simulink model "PubIfDecisionTOS_MDL"  (R2020b)
settings: configuration reference "DspaceConfig" (kept outside this file)
PostLoadFcn:
  | if any(exist('dsrtsu_mdlpostloadfcn', 'file') ~= 0), dsrtsu_mdlpostloadfcn('Execute', bdroot); end
InitFcn:
  | , if any(exist('dsmpb_private', 'file') ~= 0), dsmpb_private('dsmpb_mdlclblib', 'Init', bdroot); end,
undefined symbols (not defined in the file or in its folder): C_TOS_ACCEgoRAxletoFbumplength_m, C_TOS_ACCTargetFront_Flag, C_TOS_AEBJAPedObjDxThre_Val, C_TOS_AEBJAPedObjDyThre_Val, C_TOS_AEBJATargetSize_Val, C_TOS_AEBJAVehObjDxThre_Val, C_TOS_AEBJAVehObjDyThre_Val, C_TOS_AEBJuncPedTargetSize_Val, C_TOS_AEBLatObjDxThre_Val, C_TOS_AEBLatPedDyThre_Val, C_TOS_AEBLatTargetSize_Val, C_TOS_AEBLongTargetInEgoFront_Flag, C_TOS_axAbsGround_Parameter, C_TOS_CameraConfirmedFlag, C_TOS_CNsubjWidth, C_TOS_CurrentLaneCoreMinWidth_Val, C_TOS_CutInProb_Val_Zero, C_TOS_CutOutProb_Val_Zero, C_TOS_D2R_Val, C_TOS_DefaultValueObjectToCenterLine_dy, C_TOS_EgoCarWidth_Val, C_TOS_EgoDxRefPoint_m, C_TOS_EgoRAxletoFbumplength_m, C_TOS_HalfWidthVehicle_Con, C_TOS_HWA_CurrentLaneFlag, C_TOS_HWA_LeftLaneFlag, C_TOS_HWA_MovingDir_Vaild, C_TOS_HWA_MovState_Vaild, C_TOS_HWA_RightLaneFlag, C_TOS_LaneLineCourseErrorFront, C_TOS_LaneLineCourseErrorRear, C_TOS_MotorbikeDefaultWidth_m, C_TOS_NumberOfEffectiveTargets, C_TOS_Obj_Age_Val, C_TOS_Objdx_Constraint_Val, C_TOS_ObjectDefaultWidth_m, C_TOS_ObjInCurrentLane_Val, C_TOS_ObjInCurrentLaneValid, C_TOS_ObjInLeftLaneValid, C_TOS_ObjInRightLaneValid, C_TOS_ObjNotInCurrentLane_Val, C_TOS_ObjNotREElementType, C_TOS_ObjPredictDis_dy_ConstantVal_Zeros, C_TOS_ObjToCenterLine_ConstantVal_Zeros, C_TOS_OFMObjIDInvilad_Val, C_TOS_PIL_LatDisCons_Val_zero, C_TOS_PIL_ObjectCutInFlag_b, C_TOS_PIL_ObjectCutOutFlag_b, C_TOS_PIL_ObjLaneProb_al_Val, C_TOS_PP_ObjFusType_FC_Confirm_b, C_TOS_PP_ObjFusType_FC_FR_Confirm_b, C_TOS_PP_ObjFusType_FR_Confirm_b, C_TOS_RE_80BoolDefault_Val, C_TOS_RE_80Single181Default_Val, C_TOS_RE_80Single255Default_Val, C_TOS_RE_80Uint8Default_Val, C_TOS_RE_D2R, C_TOS_RE_D_180_Val, C_TOS_RE_InvalidObjectID_Val, C_TOS_RE_InvalidTargetChainDir_Val ... (+142)
libraries: simulink x1650, TOS_LIB x361, canfdmsglib x14
(part 30 of 69)

== system PubIfDecisionTOS_MDL/TOS_20201112/TOS_2012080320/TOS/LC_LCKie_ELK/TOS_HWA/CurrentLane/HWA_CurrentLane_Target/HWA_CLF_Target_1 ==
  HWA_CLF_Trg_1_Index : Inport
  Object_ID : Inport  Port=2
  Object_Fus_Type : Inport  Port=3
  object_MovingState : Inport  Port=4
  PP_ObjMovingDirSignalProcessing : Inport  Port=5
  Object_HeadingAngle : Inport  Port=6
  Object_DX : Inport  Port=7
  TOS_TLJ_SameLaneConfirm_Flag : Inport  Port=8
  Object_Type : Inport  Port=9
  Object_ObstacleProb : Inport  Port=10
  Object_DY : Inport  Port=11
  PP_ObjFusType_FC_FR_Confirm : Inport  Port=12
  PP_ObjFusType_FR_Confirm : Inport  Port=13
  PP_ObjFusType_FC_Confirm : Inport  Port=14
  Object_VX : Inport  Port=15
  Object_VY : Inport  Port=16
  VIE_EgoVelocity : Inport  Port=17
  SteerWheelAng : Inport  Port=18
  PIL_OverlapRatio : Inport  Port=19
  HWA_CLF_Target_ID_K1 : Inport  Port=20
  HWA_CLF_Target_ID_K2 : Inport  Port=21
  HWA_CLF_Target_MovState_K1 : Inport  Port=22
  HWA_CLF_Target_MovState_K2 : Inport  Port=23
  LM_LR_Line04_dDisStart : Inport  Port=24
  LM_LR_Line04_dDisEnd : Inport  Port=25
  LM_LR_Line05_dDisStart : Inport  Port=26
  LM_LR_Line05_dDisEnd : Inport  Port=27
  LM_LR_Line06_dDisStart : Inport  Port=28
  LM_LR_Line06_dDisEnd : Inport  Port=29
  LM_LR_Line04_pC2 : Inport  Port=30
  LM_LR_Line05_pC2 : Inport  Port=31
  LM_LR_Line06_pC2 : Inport  Port=32
  LM_LR_Line04_fCamValid : Inport  Port=33
  LM_LR_Line05_fCamValid : Inport  Port=34
  LM_LR_Line06_fCamValid : Inport  Port=35
  LM_LR_Line04_pC0 : Inport  Port=36
  LM_RL_Line04_pC0 : Inport  Port=37
  Compare To Constant : simulink/Logic and Bit Operations/Compare To Constant  relop===  const=C_TOS_OFMObjIDInvilad_Val  OutDataTypeStr=boolean
      settings: AttributesFormatString=C_TOS_OFMObjIDInvilad_Val = 0
  Constant1 : Constant  Value=0  OutDataTypeStr=uint8
  HWA_CLF_Target : Subsystem
  HWA_CLF_TargetDefault : Subsystem  TreatAsAtomicUnit=on
  If : If  IfExpression=u1 ~= 0
  Merge{,1..18} (19 alike) : Merge
  Selector3 : Selector  InputPortWidth=3  IndexOptions=Index vector (dialog)  Indices=1  OutputSizes=1
  Switch1 : Switch  Criteria=u2 ~= 0
  HWA_CLF_Target_1_Index : Outport
  HWA_CLF_Target_FusionType_ObserVale : Outport  Port=2
  HWA_CLF_Target_TrgMovDir_ObserVale : Outport  Port=3
  HWA_CLF_Target_TargetDxConfirm_ObserVale : Outport  Port=4
  HWA_CLF_Target_ObjType_ObserVale : Outport  Port=5
  HWA_CLF_Target_ObstacleProb_ObserVale : Outport  Port=6
  HWA_CLF_Target_DyConfirm_ObserVale : Outport  Port=7
  HWA_CLF_Target_TrgMovDirFlag_1_ObserVale : Outport  Port=8
  HWA_CLF_Target_TrgMovDirFlag_2_ObserVale : Outport  Port=9
  HWA_CLF_Target_TrgMovDirFlag_3_ObserVale : Outport  Port=10
  HWA_CLF_Target_TrgMovDirFlag_4_ObserVale : Outport  Port=11
  HWA_CLF_Target_TrgMovDirFlag_5_ObserVale : Outport  Port=12
  HWA_CLF_Target_TrgMovDirFlag_6_ObserVale : Outport  Port=13
  HWA_CLF_Target_DyConfirm_1_ObserVale : Outport  Port=14
  HWA_CLF_Target_DyConfirm_2_ObserVale : Outport  Port=15
  HWA_CLF_Target_DyConfirm_3_ObserVale : Outport  Port=16
  HWA_CLF_Target_DyConfirm_4_OverlapRatio_ObserVale : Outport  Port=17
  HWA_CLF_Target_DyConfirm_5_OverlapConfirm_ObserVale : Outport  Port=18
  HWA_CLF_Target_DyConfirm_ALL_6_ObserVale : Outport  Port=19
  wires:
  LM_RL_Line04_pC0/1 -> HWA_CLF_Target/37(LM_RL_Line04_pC0)  "LM_RL_Line04_pC0"
  LM_LR_Line04_pC0/1 -> HWA_CLF_Target/36(LM_LR_Line04_pC0)  "LM_LR_Line04_pC0"
  HWA_CLF_TargetDefault/19(HWA_CLF_Target_DyConfirm_ALL_6_ObserVale) -> Merge18/1
  Merge18/1 -> HWA_CLF_Target_DyConfirm_ALL_6_ObserVale/1
  HWA_CLF_Target/19(HWA_CLF_Target_DyConfirm_ALL_6_ObserVale) -> Merge18/2
  HWA_CLF_TargetDefault/18(HWA_CLF_Target_DyConfirm_5_OverlapConfirm_ObserVale) -> Merge17/1
  HWA_CLF_TargetDefault/17(HWA_CLF_Target_DyConfirm_4_OverlapRatio_ObserVale) -> Merge15/1
  HWA_CLF_TargetDefault/16(HWA_CLF_Target_DyConfirm_3_ObserVale) -> Merge14/1
  HWA_CLF_TargetDefault/15(HWA_CLF_Target_DyConfirm_2_ObserVale) -> Merge13/1
  HWA_CLF_TargetDefault/14(HWA_CLF_Target_DyConfirm_1_ObserVale) -> Merge16/1
  HWA_CLF_TargetDefault/13(HWA_CLF_Target_TrgMovDirFlag_6_ObserVale) -> Merge8/1
  HWA_CLF_TargetDefault/12(HWA_CLF_Target_TrgMovDirFlag_5_ObserVale) -> Merge12/1
  HWA_CLF_TargetDefault/11(HWA_CLF_Target_TrgMovDirFlag_4_ObserVale) -> Merge11/1
  HWA_CLF_TargetDefault/10(HWA_CLF_Target_TrgMovDirFlag_3_ObserVale) -> Merge10/1
  HWA_CLF_TargetDefault/9(HWA_CLF_Target_TrgMovDirFlag_2_ObserVale) -> Merge9/1
  HWA_CLF_TargetDefault/8(HWA_CLF_Target_TrgMovDirFlag_1_ObserVale) -> Merge7/1
  HWA_CLF_TargetDefault/7(HWA_CLF_Target_DyConfirm_ObserVale) -> Merge6/1
  HWA_CLF_TargetDefault/6(HWA_CLF_Target_ObstacleProb_ObserVale) -> Merge5/1
  HWA_CLF_TargetDefault/5(HWA_CLF_Target_ObjType_ObserVale) -> Merge4/1
  HWA_CLF_TargetDefault/4(HWA_CLF_Target_TargetDxConfirm_ObserVale) -> Merge3/1
  HWA_CLF_TargetDefault/3(HWA_CLF_Target_TrgMovDir_ObserVale) -> Merge2/1
  HWA_CLF_TargetDefault/2(HWA_CLF_Target_FusionType_ObserVale) -> Merge1/1
  HWA_CLF_TargetDefault/1(HWA_CLF_Target_2_TargeConfirm) -> Merge/1
  HWA_CLF_Target/18(HWA_CLF_Target_DyConfirm_5_OverlapConfirm_ObserVale) -> Merge17/2
  Merge17/1 -> HWA_CLF_Target_DyConfirm_5_OverlapConfirm_ObserVale/1
  LM_LR_Line06_fCamValid/1 -> HWA_CLF_Target/35(LM_LR_Line06_fCamValid)
  LM_LR_Line05_fCamValid/1 -> HWA_CLF_Target/34(LM_LR_Line05_fCamValid)
  LM_LR_Line04_fCamValid/1 -> HWA_CLF_Target/33(LM_LR_Line04_fCamValid)
  LM_LR_Line06_pC2/1 -> HWA_CLF_Target/32(LM_LR_Line06_pC2)
  LM_LR_Line05_pC2/1 -> HWA_CLF_Target/31(LM_LR_Line05_pC2)
  LM_LR_Line04_pC2/1 -> HWA_CLF_Target/30(LM_LR_Line04_pC2)
  LM_LR_Line06_dDisEnd/1 -> HWA_CLF_Target/29(LM_LR_Line06_dDisEnd)
  LM_LR_Line06_dDisStart/1 -> HWA_CLF_Target/28(LM_LR_Line06_dDisStart)
  LM_LR_Line05_dDisEnd/1 -> HWA_CLF_Target/27(LM_LR_Line05_dDisEnd)
  LM_LR_Line05_dDisStart/1 -> HWA_CLF_Target/26(LM_LR_Line05_dDisStart)
  LM_LR_Line04_dDisEnd/1 -> HWA_CLF_Target/25(LM_LR_Line04_dDisEnd)
  LM_LR_Line04_dDisStart/1 -> HWA_CLF_Target/24(LM_LR_Line04_dDisStart)
  HWA_CLF_Target/14(HWA_CLF_Target_DyConfirm_1_ObserVale) -> Merge16/2
  Merge16/1 -> HWA_CLF_Target_DyConfirm_1_ObserVale/1
  Switch1/1 -> HWA_CLF_Target_1_Index/1
  Selector3/1 -> [HWA_CurrentFront_Target_1_Index], Compare To Constant/1
  Merge15/1 -> HWA_CLF_Target_DyConfirm_4_OverlapRatio_ObserVale/1
  Merge14/1 -> HWA_CLF_Target_DyConfirm_3_ObserVale/1
  Merge13/1 -> HWA_CLF_Target_DyConfirm_2_ObserVale/1
  HWA_CLF_Target/17(HWA_CLF_Target_DyConfirm_4_OverlapRatio_ObserVale) -> Merge15/2
  HWA_CLF_Target/16(HWA_CLF_Target_DyConfirm_3_ObserVale) -> Merge14/2
  HWA_CLF_Target/15(HWA_CLF_Target_DyConfirm_2_ObserVale) -> Merge13/2
  HWA_CLF_Target/12(HWA_CLF_Target_TrgMovDirFlag_5_ObserVale) -> Merge12/2
  HWA_CLF_Target/11(HWA_CLF_Target_TrgMovDirFlag_4_ObserVale) -> Merge11/2
  HWA_CLF_Target/10(HWA_CLF_Target_TrgMovDirFlag_3_ObserVale) -> Merge10/2
  HWA_CLF_Target/9(HWA_CLF_Target_TrgMovDirFlag_2_ObserVale) -> Merge9/2
  Merge12/1 -> HWA_CLF_Target_TrgMovDirFlag_5_ObserVale/1
  Merge11/1 -> HWA_CLF_Target_TrgMovDirFlag_4_ObserVale/1
  Merge10/1 -> HWA_CLF_Target_TrgMovDirFlag_3_ObserVale/1
  Merge9/1 -> HWA_CLF_Target_TrgMovDirFlag_2_ObserVale/1
  Merge8/1 -> HWA_CLF_Target_TrgMovDirFlag_6_ObserVale/1
  HWA_CLF_Target/13(HWA_CLF_Target_TrgMovDirFlag_6_ObserVale) -> Merge8/2
  Object_ID/1 -> HWA_CLF_Target/23(ObjectID)
  HWA_CLF_Target_MovState_K2/1 -> HWA_CLF_Target/22(HWA_CLF_Target_Target_MovState_K2)
  HWA_CLF_Target_MovState_K1/1 -> HWA_CLF_Target/21(HWA_CLF_Target_Target_MovState_K1)
  HWA_CLF_Target_ID_K2/1 -> HWA_CLF_Target/20(HWA_CLF_Target_Target_ID_K2)
  HWA_CLF_Target_ID_K1/1 -> HWA_CLF_Target/19(HWA_CLF_Target_ID_K1)
  Merge7/1 -> HWA_CLF_Target_TrgMovDirFlag_1_ObserVale/1
  HWA_CLF_Target/8(HWA_CLF_Target_TrgMovDirFlag_1_ObserVale) -> Merge7/2
  PIL_OverlapRatio/1 -> HWA_CLF_Target/18(PIL_OverlapRatio)
  SteerWheelAng/1 -> HWA_CLF_Target/17(SteerWheelAng)
  VIE_EgoVelocity/1 -> HWA_CLF_Target/16(VIE_EgoVelocity)
  Object_VX/1 -> HWA_CLF_Target/14(Object_VX)
  Object_VY/1 -> HWA_CLF_Target/15(Object_VY)
  PP_ObjFusType_FR_Confirm/1 -> HWA_CLF_Target/12(PP_ObjFusType_FR_Confirm)
  PP_ObjFusType_FC_FR_Confirm/1 -> HWA_CLF_Target/11(PP_ObjFusType_FC_FR_Confirm)
  PP_ObjFusType_FC_Confirm/1 -> HWA_CLF_Target/13(PP_ObjFusType_FC_Confirm)
  If/2 -> HWA_CLF_Target/Action
  HWA_CLF_Target/7(HWA_CLF_Target_DyConfirm_ObserVale) -> Merge6/2
  HWA_CLF_Target/6(HWA_CLF_Target_ObstacleProb_ObserVale) -> Merge5/2
  HWA_CLF_Target/5(HWA_CLF_Target_ObjType_ObserVale) -> Merge4/2
  HWA_CLF_Target/4(HWA_CLF_Target_TargetDxConfirm_ObserVale) -> Merge3/2
  HWA_CLF_Target/3(HWA_CLF_Target_TrgMovDir_ObserVale) -> Merge2/2
  HWA_CLF_Target/2(HWA_CLF_Target_FusionType_ObserVale) -> Merge1/2
  HWA_CLF_Target/1(HWA_CLF_Target_1_TargeConfirm) -> Merge/2
  Object_DY/1 -> HWA_CLF_Target/10(Object_DY)
  Object_ObstacleProb/1 -> HWA_CLF_Target/9(Object_ObstacleProb)
  Object_Type/1 -> HWA_CLF_Target/8(Object_Type)
  TOS_TLJ_SameLaneConfirm_Flag/1 -> HWA_CLF_Target/7(TOS_TLJ_SameLaneConfirm_Flag)
  Object_DX/1 -> HWA_CLF_Target/6(Object_DX)
  Object_HeadingAngle/1 -> HWA_CLF_Target/5(Object_HeadingAngle)
  PP_ObjMovingDirSignalProcessing/1 -> HWA_CLF_Target/4(PP_ObjMovingDirSignalProcessing)
  object_MovingState/1 -> HWA_CLF_Target/3(object_MovingState)
  Object_Fus_Type/1 -> HWA_CLF_Target/2(Object_Fus_Type)
  [HWA_CurrentFront_Target_1_Index] -> HWA_CLF_Target/1(HWA_CLF_Target_1_Index)
  HWA_CLF_Trg_1_Index/1 -> Selector3/1
  Constant1/1 -> Switch1/3
  Merge/1 -> Switch1/2
  [HWA_CurrentFront_Target_1_Index] -> Switch1/1
  Merge6/1 -> HWA_CLF_Target_DyConfirm_ObserVale/1
  Merge5/1 -> HWA_CLF_Target_ObstacleProb_ObserVale/1
  Merge4/1 -> HWA_CLF_Target_ObjType_ObserVale/1
  Merge3/1 -> HWA_CLF_Target_TargetDxConfirm_ObserVale/1
  Merge2/1 -> HWA_CLF_Target_TrgMovDir_ObserVale/1
  Merge1/1 -> HWA_CLF_Target_FusionType_ObserVale/1
  Compare To Constant/1 -> If/1
  If/1 -> HWA_CLF_TargetDefault/Action

== system PubIfDecisionTOS_MDL/TOS_20201112/TOS_2012080320/TOS/LC_LCKie_ELK/TOS_HWA/CurrentLane/HWA_CurrentLane_Target/HWA_CLF_Target_2 ==
  HWA_CLF_Trg_2_Index : Inport
  Object_ID : Inport  Port=2
  Object_Fus_Type : Inport  Port=3
  object_MovingState : Inport  Port=4
  PP_ObjMovingDirSignalProcessing : Inport  Port=5
  Object_HeadingAngle : Inport  Port=6
  Object_DX : Inport  Port=7
  TOS_TLJ_SameLaneConfirm_Flag : Inport  Port=8
  Object_Type : Inport  Port=9
  Object_ObstacleProb : Inport  Port=10
  Object_DY : Inport  Port=11
  PP_ObjFusType_FC_FR_Confirm : Inport  Port=12
  PP_ObjFusType_FR_Confirm : Inport  Port=13
  PP_ObjFusType_FC_Confirm : Inport  Port=14
  Object_VX : Inport  Port=15
  Object_VY : Inport  Port=16
  VIE_EgoVelocity : Inport  Port=17
  SteerWheelAng : Inport  Port=18
  PIL_OverlapRatio : Inport  Port=19
  HWA_CLF_Target_ID_K1 : Inport  Port=20
  HWA_CLF_Target_ID_K2 : Inport  Port=21
  HWA_CLF_Target_MovState_K1 : Inport  Port=22
  HWA_CLF_Target_MovState_K2 : Inport  Port=23
  LM_LR_Line04_dDisStart : Inport  Port=24
  LM_LR_Line04_dDisEnd : Inport  Port=25
  LM_LR_Line05_dDisStart : Inport  Port=26
  LM_LR_Line05_dDisEnd : Inport  Port=27
  LM_LR_Line06_dDisStart : Inport  Port=28
  LM_LR_Line06_dDisEnd : Inport  Port=29
  LM_LR_Line04_pC2 : Inport  Port=30
  LM_LR_Line05_pC2 : Inport  Port=31
  LM_LR_Line06_pC2 : Inport  Port=32
  LM_LR_Line04_fCamValid : Inport  Port=33
  LM_LR_Line05_fCamValid : Inport  Port=34
  LM_LR_Line06_fCamValid : Inport  Port=35
  LM_LR_Line04_pC0 : Inport  Port=36
  LM_RL_Line04_pC0 : Inport  Port=37
  Compare To Constant : simulink/Logic and Bit Operations/Compare To Constant  relop===  const=C_TOS_OFMObjIDInvilad_Val  OutDataTypeStr=boolean
      settings: AttributesFormatString=C_TOS_OFMObjIDInvilad_Val = 0
  Constant1 : Constant  Value=0  OutDataTypeStr=uint8
  HWA_CLF_Target : Subsystem
  HWA_CLF_TargetDefault : Subsystem  TreatAsAtomicUnit=on
  If : If  IfExpression=u1 ~= 0
  Merge{,1..18} (19 alike) : Merge
  Selector3 : Selector  InputPortWidth=3  IndexOptions=Index vector (dialog)  Indices=[2]  OutputSizes=1
  Switch1 : Switch  Criteria=u2 ~= 0
  HWA_CLF_Target_2_Index : Outport
  HWA_CLF_Target_FusionType_ObserVale : Outport  Port=2
  HWA_CLF_Target_TrgMovDir_ObserVale : Outport  Port=3
  HWA_CLF_Target_TargetDxConfirm_ObserVale : Outport  Port=4
  HWA_CLF_Target_ObjType_ObserVale : Outport  Port=5
  HWA_CLF_Target_ObstacleProb_ObserVale : Outport  Port=6
  HWA_CLF_Target_DyConfirm_ObserVale : Outport  Port=7
  HWA_CLF_Target_TrgMovDirFlag_1_ObserVale : Outport  Port=8
  HWA_CLF_Target_TrgMovDirFlag_2_ObserVale : Outport  Port=9
  HWA_CLF_Target_TrgMovDirFlag_3_ObserVale : Outport  Port=10
  HWA_CLF_Target_TrgMovDirFlag_4_ObserVale : Outport  Port=11
  HWA_CLF_Target_TrgMovDirFlag_5_ObserVale : Outport  Port=12
  HWA_CLF_Target_TrgMovDirFlag_6_ObserVale : Outport  Port=13
  HWA_CLF_Target_DyConfirm_1_ObserVale : Outport  Port=14
  HWA_CLF_Target_DyConfirm_2_ObserVale : Outport  Port=15
  HWA_CLF_Target_DyConfirm_3_ObserVale : Outport  Port=16
  HWA_CLF_Target_DyConfirm_4_OverlapRatio_ObserVale : Outport  Port=17
  HWA_CLF_Target_DyConfirm_5_OverlapConfirm_ObserVale : Outport  Port=18
  HWA_CLF_Target_DyConfirm_ALL_6_ObserVale : Outport  Port=19
  wires:
  If/1 -> HWA_CLF_TargetDefault/Action
  Compare To Constant/1 -> If/1
  Merge1/1 -> HWA_CLF_Target_FusionType_ObserVale/1
  Merge2/1 -> HWA_CLF_Target_TrgMovDir_ObserVale/1
  Merge3/1 -> HWA_CLF_Target_TargetDxConfirm_ObserVale/1
  Merge4/1 -> HWA_CLF_Target_ObjType_ObserVale/1
  Merge5/1 -> HWA_CLF_Target_ObstacleProb_ObserVale/1
  Merge6/1 -> HWA_CLF_Target_DyConfirm_ObserVale/1
  [HWA_CurrentFront_Target_2_Index] -> Switch1/1
  Merge/1 -> Switch1/2
  Constant1/1 -> Switch1/3
  HWA_CLF_Trg_2_Index/1 -> Selector3/1
  [HWA_CurrentFront_Target_2_Index] -> HWA_CLF_Target/1(HWA_CLF_Target_2_Index)
  Object_Fus_Type/1 -> HWA_CLF_Target/2(Object_Fus_Type)
  object_MovingState/1 -> HWA_CLF_Target/3(object_MovingState)
  PP_ObjMovingDirSignalProcessing/1 -> HWA_CLF_Target/4(PP_ObjMovingDirSignalProcessing)
  Object_HeadingAngle/1 -> HWA_CLF_Target/5(Object_HeadingAngle)
  Object_DX/1 -> HWA_CLF_Target/6(Object_DX)
  TOS_TLJ_SameLaneConfirm_Flag/1 -> HWA_CLF_Target/7(TOS_TLJ_SameLaneConfirm_Flag)
  Object_Type/1 -> HWA_CLF_Target/8(Object_Type)
  Object_ObstacleProb/1 -> HWA_CLF_Target/9(Object_ObstacleProb)
  Object_DY/1 -> HWA_CLF_Target/10(Object_DY)
  HWA_CLF_Target/1(HWA_CLF_Target_2_TargeConfirm) -> Merge/2
  HWA_CLF_Target/2(HWA_CLF_Target_FusionType_ObserVale) -> Merge1/2
  HWA_CLF_Target/3(HWA_CLF_Target_TrgMovDir_ObserVale) -> Merge2/2
  HWA_CLF_Target/4(HWA_CLF_Target_TargetDxConfirm_ObserVale) -> Merge3/2
  HWA_CLF_Target/5(HWA_CLF_Target_ObjType_ObserVale) -> Merge4/2
  HWA_CLF_Target/6(HWA_CLF_Target_ObstacleProb_ObserVale) -> Merge5/2
  HWA_CLF_Target/7(HWA_CLF_Target_DyConfirm_ObserVale) -> Merge6/2
  If/2 -> HWA_CLF_Target/Action
  PP_ObjFusType_FC_Confirm/1 -> HWA_CLF_Target/13(PP_ObjFusType_FC_Confirm)
  PP_ObjFusType_FC_FR_Confirm/1 -> HWA_CLF_Target/11(PP_ObjFusType_FC_FR_Confirm)
  PP_ObjFusType_FR_Confirm/1 -> HWA_CLF_Target/12(PP_ObjFusType_FR_Confirm)
  Object_VY/1 -> HWA_CLF_Target/15(Object_VY)
  Object_VX/1 -> HWA_CLF_Target/14(Object_VX)
  VIE_EgoVelocity/1 -> HWA_CLF_Target/16(VIE_EgoVelocity)
  SteerWheelAng/1 -> HWA_CLF_Target/17(SteerWheelAng)
  PIL_OverlapRatio/1 -> HWA_CLF_Target/18(PIL_OverlapRatio)
  HWA_CLF_Target/8(HWA_CLF_Target_TrgMovDirFlag_1_ObserVale) -> Merge7/2
  Merge7/1 -> HWA_CLF_Target_TrgMovDirFlag_1_ObserVale/1
  HWA_CLF_Target_ID_K1/1 -> HWA_CLF_Target/19(HWA_CLF_Target_ID_K1)
  HWA_CLF_Target_ID_K2/1 -> HWA_CLF_Target/20(HWA_CLF_Target_Target_ID_K2)
  HWA_CLF_Target_MovState_K1/1 -> HWA_CLF_Target/21(HWA_CLF_Target_Target_MovState_K1)
  HWA_CLF_Target_MovState_K2/1 -> HWA_CLF_Target/22(HWA_CLF_Target_Target_MovState_K2)
  Object_ID/1 -> HWA_CLF_Target/23(ObjectID)
  HWA_CLF_Target/13(HWA_CLF_Target_TrgMovDirFlag_6_ObserVale) -> Merge8/2
  Merge8/1 -> HWA_CLF_Target_TrgMovDirFlag_6_ObserVale/1
  Merge9/1 -> HWA_CLF_Target_TrgMovDirFlag_2_ObserVale/1
  Merge10/1 -> HWA_CLF_Target_TrgMovDirFlag_3_ObserVale/1
  Merge11/1 -> HWA_CLF_Target_TrgMovDirFlag_4_ObserVale/1
  Merge12/1 -> HWA_CLF_Target_TrgMovDirFlag_5_ObserVale/1
  HWA_CLF_Target/9(HWA_CLF_Target_TrgMovDirFlag_2_ObserVale) -> Merge9/2
  HWA_CLF_Target/10(HWA_CLF_Target_TrgMovDirFlag_3_ObserVale) -> Merge10/2
  HWA_CLF_Target/11(HWA_CLF_Target_TrgMovDirFlag_4_ObserVale) -> Merge11/2
  HWA_CLF_Target/12(HWA_CLF_Target_TrgMovDirFlag_5_ObserVale) -> Merge12/2
  HWA_CLF_Target/15(HWA_CLF_Target_DyConfirm_2_ObserVale) -> Merge13/2
  HWA_CLF_Target/16(HWA_CLF_Target_DyConfirm_3_ObserVale) -> Merge14/2
  HWA_CLF_Target/17(HWA_CLF_Target_DyConfirm_4_OverlapRatio_ObserVale) -> Merge15/2
  Merge13/1 -> HWA_CLF_Target_DyConfirm_2_ObserVale/1
  Merge14/1 -> HWA_CLF_Target_DyConfirm_3_ObserVale/1
  Merge15/1 -> HWA_CLF_Target_DyConfirm_4_OverlapRatio_ObserVale/1
  Selector3/1 -> [HWA_CurrentFront_Target_2_Index], Compare To Constant/1
  Switch1/1 -> HWA_CLF_Target_2_Index/1
  Merge16/1 -> HWA_CLF_Target_DyConfirm_1_ObserVale/1
  HWA_CLF_Target/14(HWA_CLF_Target_DyConfirm_1_ObserVale) -> Merge16/2
  LM_LR_Line04_dDisStart/1 -> HWA_CLF_Target/24(LM_LR_Line04_dDisStart)
  LM_LR_Line04_dDisEnd/1 -> HWA_CLF_Target/25(LM_LR_Line04_dDisEnd)
  LM_LR_Line05_dDisStart/1 -> HWA_CLF_Target/26(LM_LR_Line05_dDisStart)
  LM_LR_Line05_dDisEnd/1 -> HWA_CLF_Target/27(LM_LR_Line05_dDisEnd)
  LM_LR_Line06_dDisStart/1 -> HWA_CLF_Target/28(LM_LR_Line06_dDisStart)
  LM_LR_Line06_dDisEnd/1 -> HWA_CLF_Target/29(LM_LR_Line06_dDisEnd)
  LM_LR_Line04_pC2/1 -> HWA_CLF_Target/30(LM_LR_Line04_pC2)
  LM_LR_Line05_pC2/1 -> HWA_CLF_Target/31(LM_LR_Line05_pC2)
  LM_LR_Line06_pC2/1 -> HWA_CLF_Target/32(LM_LR_Line06_pC2)
  LM_LR_Line04_fCamValid/1 -> HWA_CLF_Target/33(LM_LR_Line04_fCamValid)
  LM_LR_Line05_fCamValid/1 -> HWA_CLF_Target/34(LM_LR_Line05_fCamValid)
  LM_LR_Line06_fCamValid/1 -> HWA_CLF_Target/35(LM_LR_Line06_fCamValid)
  Merge17/1 -> HWA_CLF_Target_DyConfirm_5_OverlapConfirm_ObserVale/1
  HWA_CLF_Target/18(HWA_CLF_Target_DyConfirm_5_OverlapConfirm_ObserVale) -> Merge17/2
  HWA_CLF_TargetDefault/1(HWA_CLF_Target_2_TargeConfirm) -> Merge/1
  HWA_CLF_TargetDefault/2(HWA_CLF_Target_FusionType_ObserVale) -> Merge1/1
  HWA_CLF_TargetDefault/3(HWA_CLF_Target_TrgMovDir_ObserVale) -> Merge2/1
  HWA_CLF_TargetDefault/4(HWA_CLF_Target_TargetDxConfirm_ObserVale) -> Merge3/1
  HWA_CLF_TargetDefault/5(HWA_CLF_Target_ObjType_ObserVale) -> Merge4/1
  HWA_CLF_TargetDefault/6(HWA_CLF_Target_ObstacleProb_ObserVale) -> Merge5/1
  HWA_CLF_TargetDefault/7(HWA_CLF_Target_DyConfirm_ObserVale) -> Merge6/1
  HWA_CLF_TargetDefault/8(HWA_CLF_Target_TrgMovDirFlag_1_ObserVale) -> Merge7/1
  HWA_CLF_TargetDefault/9(HWA_CLF_Target_TrgMovDirFlag_2_ObserVale) -> Merge9/1
  HWA_CLF_TargetDefault/10(HWA_CLF_Target_TrgMovDirFlag_3_ObserVale) -> Merge10/1
  HWA_CLF_TargetDefault/11(HWA_CLF_Target_TrgMovDirFlag_4_ObserVale) -> Merge11/1
  HWA_CLF_TargetDefault/12(HWA_CLF_Target_TrgMovDirFlag_5_ObserVale) -> Merge12/1
  HWA_CLF_TargetDefault/13(HWA_CLF_Target_TrgMovDirFlag_6_ObserVale) -> Merge8/1
  HWA_CLF_TargetDefault/14(HWA_CLF_Target_DyConfirm_1_ObserVale) -> Merge16/1
  HWA_CLF_TargetDefault/15(HWA_CLF_Target_DyConfirm_2_ObserVale) -> Merge13/1
  HWA_CLF_TargetDefault/16(HWA_CLF_Target_DyConfirm_3_ObserVale) -> Merge14/1
  HWA_CLF_TargetDefault/17(HWA_CLF_Target_DyConfirm_4_OverlapRatio_ObserVale) -> Merge15/1
  HWA_CLF_TargetDefault/18(HWA_CLF_Target_DyConfirm_5_OverlapConfirm_ObserVale) -> Merge17/1
  HWA_CLF_Target/19(HWA_CLF_Target_DyConfirm_ALL_6_ObserVale) -> Merge18/2
  Merge18/1 -> HWA_CLF_Target_DyConfirm_ALL_6_ObserVale/1
  HWA_CLF_TargetDefault/19(HWA_CLF_Target_DyConfirm_ALL_6_ObserVale) -> Merge18/1
  LM_LR_Line04_pC0/1 -> HWA_CLF_Target/36(LM_LR_Line04_pC0)  "LM_LR_Line04_pC0"
  LM_RL_Line04_pC0/1 -> HWA_CLF_Target/37(LM_RL_Line04_pC0)  "LM_RL_Line04_pC0"

== system PubIfDecisionTOS_MDL/TOS_20201112/TOS_2012080320/TOS/LC_LCKie_ELK/TOS_HWA/CurrentLane/HWA_CurrentLane_Target/HWA_CLF_Target_3 ==
  HWA_CLF_Target_3 : Inport
  PP_ObjMovingDirSignalProcessing : Inport  Port=2
  Object_VX : Inport  Port=3
  Object_VY : Inport  Port=4
  Object_Type : Inport  Port=5
  Object_MovingState : Inport  Port=6
  TOS_TLJ_SameLaneConfirm_Flag : Inport  Port=7
  Object_DX : Inport  Port=8
  Object_DY : Inport  Port=9
  Object_Fus_Type : Inport  Port=10
  Object_HeadingAngle : Inport  Port=11
  PP_ObjFusType_FC_FR_Confirm : Inport  Port=12
  PP_ObjFusType_FR_Confirm : Inport  Port=13
  PP_ObjFusType_FC_Confirm : Inport  Port=14
  VIE_EgoVelocity : Inport  Port=15
  Compare To Constant : simulink/Logic and Bit Operations/Compare To Constant  relop===  const=C_TOS_OFMObjIDInvilad_Val  OutDataTypeStr=boolean
      settings: AttributesFormatString=C_TOS_OFMObjIDInvilad_Val = 0
  Constant1 : Constant  Value=0  OutDataTypeStr=uint8
  HWA_CLR_Target : Subsystem
  HWA_CLR_Target_Default : Subsystem  TreatAsAtomicUnit=on
  If : If  IfExpression=u1 ~= 0
  Merge{1,7..9,11..12} (6 alike) : Merge
  Selector3 : Selector  InputPortWidth=3  IndexOptions=Index vector (dialog)  Indices=3  OutputSizes=1
  Switch1 : Switch  Criteria=u2 ~= 0
  HWA_CLR_Target_3_Index : Outport
  HWA_CLR_Target_3_MovState_ObserVale : Outport  Port=2
  HWA_CLR_Target_3_ObjType_ObserVale : Outport  Port=3
  HWA_CLR_Target_3_InCurrentLane_Flag_ObserVale : Outport  Port=4
  HWA_CLR_Target_3_TargetMovingDir_ObserVale : Outport  Port=5
  HWA_CLR_Target_3_DyConfirm_ObserVale : Outport  Port=6
  wires:
  Object_DY/1 -> HWA_CLR_Target/9(Object_DY)  "Object_DY"
  HWA_CLR_Target/1(HWA_CLR_Target_3_TargeConfirm) -> Merge1/2
  VIE_EgoVelocity/1 -> HWA_CLR_Target/15(VIE_EgoVelocity)
  PP_ObjFusType_FR_Confirm/1 -> HWA_CLR_Target/13(PP_ObjFusType_FR_Confirm)
  PP_ObjFusType_FC_FR_Confirm/1 -> HWA_CLR_Target/12(PP_ObjFusType_FC_FR_Confirm)
  PP_ObjFusType_FC_Confirm/1 -> HWA_CLR_Target/14(PP_ObjFusType_FC_Confirm)
  [HWA_CLR_Target_3_Index] -> HWA_CLR_Target/1(HWA_CurrentLane_ObjIndex)
  [HWA_CLR_Target_3_Index] -> Switch1/1
  Constant1/1 -> Switch1/3
  Switch1/1 -> HWA_CLR_Target_3_Index/1
  HWA_CLF_Target_3/1 -> Selector3/1
  Object_HeadingAngle/1 -> HWA_CLR_Target/11(Object_HeadingAngle)  "Object_HeadingAngle"
  Object_Fus_Type/1 -> HWA_CLR_Target/10(Object_Fus_Type)
  Object_DX/1 -> HWA_CLR_Target/8(Object_DX)  "Object_DX"
  TOS_TLJ_SameLaneConfirm_Flag/1 -> HWA_CLR_Target/7(TOS_TLJ_SameLaneConfirm_Flag)
  Object_MovingState/1 -> HWA_CLR_Target/6(object_MovingState)
  Object_Type/1 -> HWA_CLR_Target/5(Object_Type)
  Object_VY/1 -> HWA_CLR_Target/4(Object_VY)
  Object_VX/1 -> HWA_CLR_Target/3(Object_VX)
  PP_ObjMovingDirSignalProcessing/1 -> HWA_CLR_Target/2(PP_ObjMovingDirSignalProcessing)
  If/2 -> HWA_CLR_Target/Action
  Compare To Constant/1 -> If/1
  If/1 -> HWA_CLR_Target_Default/Action
  Selector3/1 -> Compare To Constant/1, [HWA_CLR_Target_3_Index]
  HWA_CLR_Target/6(HWA_CLR_Target_3_DyConfirm_ObserVale) -> Merge11/2
  HWA_CLR_Target/2(HWA_CLR_Target_3_MovState_ObserVale) -> Merge7/2
  HWA_CLR_Target/3(HWA_CLR_Target_3_ObjType_ObserVale) -> Merge12/2
  HWA_CLR_Target/4(HWA_CLR_Target_3_InCurrentLane_Flag_ObserVale) -> Merge8/2
  HWA_CLR_Target/5(HWA_CLR_Target_3_TargetMovingDir_ObserVale) -> Merge9/2
  HWA_CLR_Target_Default/1(HWA_CLR_Target_3_TargeConfirm) -> Merge1/1
  HWA_CLR_Target_Default/2(HWA_CLR_Target_3_MovState_ObserVale) -> Merge7/1
  HWA_CLR_Target_Default/3(HWA_CLR_Target_3_ObjType_ObserVale) -> Merge12/1
  HWA_CLR_Target_Default/4(HWA_CLR_Target_3_InCurrentLane_Flag_ObserVale) -> Merge8/1
  HWA_CLR_Target_Default/5(HWA_CLR_Target_3_TargetMovingDir_ObserVale) -> Merge9/1
  HWA_CLR_Target_Default/6(HWA_CLR_Target_3_DyConfirm_ObserVale) -> Merge11/1
  Merge1/1 -> Switch1/2
  Merge7/1 -> HWA_CLR_Target_3_MovState_ObserVale/1
  Merge12/1 -> HWA_CLR_Target_3_ObjType_ObserVale/1
  Merge8/1 -> HWA_CLR_Target_3_InCurrentLane_Flag_ObserVale/1
  Merge9/1 -> HWA_CLR_Target_3_TargetMovingDir_ObserVale/1
  Merge11/1 -> HWA_CLR_Target_3_DyConfirm_ObserVale/1

== system PubIfDecisionTOS_MDL/TOS_20201112/TOS_2012080320/TOS/LC_LCKie_ELK/TOS_HWA/CurrentLane/HWA_CurrentLane_Target/Subsystem ==
  HWA_CLF_Target_1_Index : Inport
  HWA_CLF_Target_2_Index : Inport  Port=2
  HWA_CLR_Target_3_Index : Inport  Port=3
  Constant2 : Constant  Value=0  OutDataTypeStr=uint8
  Constant3 : Constant  Value=0  OutDataTypeStr=uint8
  Constant4 : Constant  Value=C_TOS_ObjInCurrentLaneValid  OutDataTypeStr=uint8
      settings: AttributesFormatString=C_TOS_ObjInCurrentLaneValid = 1
  Constant5 : Constant  Value=C_TOS_ObjInCurrentLaneValid  OutDataTypeStr=uint8
      settings: AttributesFormatString=C_TOS_ObjInCurrentLaneValid = 1
  Constant6 : Constant  Value=0  OutDataTypeStr=uint8
  Constant7 : Constant  Value=C_TOS_ObjInCurrentLaneValid  OutDataTypeStr=uint8
      settings: AttributesFormatString=C_TOS_ObjInCurrentLaneValid = 1
  Switch1 : Switch  Criteria=u2 ~= 0
  Switch2 : Switch  Criteria=u2 ~= 0
  Switch3 : Switch  Criteria=u2 ~= 0
  Vector Concatenate2 : Concatenate  NumInputs=3
  Out1 : Outport
  wires:
  Constant2/1 -> Switch2/3
  Switch2/1 -> Vector Concatenate2/1
  Constant7/1 -> Switch3/1
  Switch1/1 -> Vector Concatenate2/2
  Switch3/1 -> Vector Concatenate2/3
  Constant6/1 -> Switch3/3
  Constant5/1 -> Switch2/1
  Constant3/1 -> Switch1/3
  HWA_CLF_Target_1_Index/1 -> Switch2/2
  Constant4/1 -> Switch1/1
  HWA_CLR_Target_3_Index/1 -> Switch3/2
  HWA_CLF_Target_2_Index/1 -> Switch1/2
  Vector Concatenate2/1 -> Out1/1

== system PubIfDecisionTOS_MDL/TOS_20201112/TOS_2012080320/TOS/LC_LCKie_ELK/TOS_HWA/CurrentLane/HWA_Object_PreConfirm/TOS_HWA_CurrentLaneFront_TargPreConfirm ==
  PP_ObjFusType_FC_FR_Confirm : Inport  Partition=on  PartitionDimension=1  PartitionWidth=1  PartitionOffset=0
  PP_ObjFusType_FR_Confirm : Inport  Port=2  Partition=on  PartitionDimension=1  PartitionWidth=1  PartitionOffset=0
  PP_ObjFusType_FC_Confirm : Inport  Port=3  Partition=on  PartitionDimension=1  PartitionWidth=1  PartitionOffset=0
  Object_ID : Inport  Port=4  OutDataTypeStr=uint8  Partition=on  PartitionDimension=1  PartitionWidth=1  PartitionOffset=0
  Obj_MovingState : Inport  Port=5  Partition=on  PartitionDimension=1  PartitionWidth=1  PartitionOffset=0
  Obj_Dx : Inport  Port=6  Partition=on  PartitionDimension=1  PartitionWidth=1  PartitionOffset=0
  Object_ObstacleProb : Inport  Port=7  Partition=on  PartitionDimension=1  PartitionWidth=1  PartitionOffset=0
  Object_DY : Inport  Port=8  Partition=on  PartitionDimension=1  PartitionWidth=1  PartitionOffset=0
  Object_ObjType : Inport  Port=9  Partition=on  PartitionDimension=1  PartitionWidth=1  PartitionOffset=0
  TOS_TLJ_SameLaneConfirm_Flag : Inport  Port=10  Partition=on  PartitionDimension=1  PartitionWidth=1  PartitionOffset=0
  LM_LR_Line04_fCamValid : Inport  Port=11
  LM_LR_Line05_fCamValid : Inport  Port=12
  LM_LR_Line06_fCamValid : Inport  Port=13
  TOS_HWA_CurrentFront_Target_2_ID_K1 : Inport  Port=14
  TOS_HWA_Dx_K1 : Inport  Port=15
  PIL_OverlapRatio : Inport  Port=16  Partition=on  PartitionDimension=1  PartitionWidth=1  PartitionOffset=0
  PIL_OverlapRatio_K1 : Inport  Port=17  Partition=on  PartitionDimension=1  PartitionWidth=1  PartitionOffset=0
  PIL_OverlapRatio_K2 : Inport  Port=18  Partition=on  PartitionDimension=1  PartitionWidth=1  PartitionOffset=0
  LM_LR_Line04_dDisStart : Inport  Port=19
  LM_LR_Line04_dDisEnd : Inport  Port=20
  LM_LR_Line05_dDisStart : Inport  Port=21
  LM_LR_Line05_dDisEnd : Inport  Port=22
  LM_LR_Line06_dDisStart : Inport  Port=23
  LM_LR_Line06_dDisEnd : Inport  Port=24
  Compare To Constant : simulink/Logic and Bit Operations/Compare To Constant  relop=~=  const=C_TOS_OFMObjIDInvilad_Val  OutDataTypeStr=boolean
      settings: AttributesFormatString=C_TOS_OFMObjIDInvilad_Val = 0
  Compare To Constant1 : simulink/Logic and Bit Operations/Compare To Constant  relop=>=  const=single(0)  OutDataTypeStr=boolean
      settings: AttributesFormatString=dx >= single(0)
  Compare To Constant2 : simulink/Logic and Bit Operations/Compare To Constant  relop=<  const=single(0)  OutDataTypeStr=boolean
      settings: AttributesFormatString=dx >= single(0)
  Default : Subsystem  TreatAsAtomicUnit=on
  For Each : ForEach  DisableCoverage=on
  If : If  NumInputs=2  IfExpression=u1 == 1  ElseIfExpressions=u2 == 1
  Logical Operator1 : Logic  AllPortsSameDT=off  OutDataTypeStr=boolean
  Logical Operator3 : Logic  AllPortsSameDT=off  OutDataTypeStr=boolean
  Merge{,1..9} (10 alike) : Merge  Inputs=3
  TOS_HWA_CurrentLaneFront_TargPreConfirm : Subsystem
  TOS_HWA_CurrentLaneRear_TargPreConfirmDefault : Subsystem  TreatAsAtomicUnit=on
  TOS_HWA_TargetPre_Filt_Flag : Outport  ConcatenationDimension=1
  TOS_HWA_TargetPre_1_ConditionFlag_ObserVale : Outport  Port=2  ConcatenationDimension=1
  TOS_HWA_TargetPre_FusionTypeFlag_ObserVale : Outport  Port=3  ConcatenationDimension=1
  TOS_HWA_TargetPre_PassedbyTarget_Flag_ObserVale : Outport  Port=4  ConcatenationDimension=1
  TOS_HWA_TargetPre_FenceFlag_ObserVale : Outport  Port=5  ConcatenationDimension=1
  TOS_HWA_TargetPre_ObjType_ObserVale : Outport  Port=6  ConcatenationDimension=1
  TOS_HWA_TargetPre_OverlapThre_Val_ObserVale : Outport  Port=7  ConcatenationDimension=1
  TOS_HWA_TargetPre_SameLane_Flag : Outport  Port=8  ConcatenationDimension=1
  TOS_HWA_TargetPre_2_OverlapThre_ObserVale : Outport  Port=9  ConcatenationDimension=1
  TOS_HWA_TargetPre_3_SameLane_Flag_ObserVale : Outport  Port=10  ConcatenationDimension=1
  wires:
  PP_ObjFusType_FC_FR_Confirm/1 -> TOS_HWA_CurrentLaneFront_TargPreConfirm/2(PP_ObjFusType_FC_FR_Confirm)
  PP_ObjFusType_FR_Confirm/1 -> TOS_HWA_CurrentLaneFront_TargPreConfirm/3(PP_ObjFusType_FR_Confirm)
  Compare To Constant/1 -> Logical Operator1/1, Logical Operator3/1
  Object_ID/1 -> Compare To Constant/1, [Object_ID]
  If/1 -> TOS_HWA_CurrentLaneFront_TargPreConfirm/Action
  PP_ObjFusType_FC_Confirm/1 -> TOS_HWA_CurrentLaneFront_TargPreConfirm/4(PP_ObjFusType_FC_Confirm)
  Obj_MovingState/1 -> TOS_HWA_CurrentLaneFront_TargPreConfirm/5(Obj_MovingState)
  Obj_Dx/1 -> [Obj_Dx], TOS_HWA_CurrentLaneFront_TargPreConfirm/6(Obj_Dx)
  Object_ObstacleProb/1 -> TOS_HWA_CurrentLaneFront_TargPreConfirm/7(Object_ObstacleProb)
  Object_DY/1 -> TOS_HWA_CurrentLaneFront_TargPreConfirm/8(Object_DY)
  TOS_HWA_CurrentFront_Target_2_ID_K1/1 -> TOS_HWA_CurrentLaneFront_TargPreConfirm/14(TOS_HWA_ID_K1)
  TOS_HWA_Dx_K1/1 -> TOS_HWA_CurrentLaneFront_TargPreConfirm/15(TOS_HWA_Dx_K1)
  [Object_ID] -> TOS_HWA_CurrentLaneFront_TargPreConfirm/1(Object_ID)
  Object_ObjType/1 -> TOS_HWA_CurrentLaneFront_TargPreConfirm/9(Object_ObjType)
  PIL_OverlapRatio/1 -> TOS_HWA_CurrentLaneFront_TargPreConfirm/16(PIL_OverlapRatio)
  TOS_TLJ_SameLaneConfirm_Flag/1 -> TOS_HWA_CurrentLaneFront_TargPreConfirm/10(TOS_TLJ_SameLaneConfirm_Flag)
  PIL_OverlapRatio_K1/1 -> TOS_HWA_CurrentLaneFront_TargPreConfirm/17(PIL_OverlapRatio_K1)
  PIL_OverlapRatio_K2/1 -> TOS_HWA_CurrentLaneFront_TargPreConfirm/18(PIL_OverlapRatio_K2)
  LM_LR_Line04_fCamValid/1 -> TOS_HWA_CurrentLaneFront_TargPreConfirm/11(LM_LR_Line04_fCamValid)
  LM_LR_Line05_fCamValid/1 -> TOS_HWA_CurrentLaneFront_TargPreConfirm/12(LM_LR_Line05_fCamValid)
  LM_LR_Line06_fCamValid/1 -> TOS_HWA_CurrentLaneFront_TargPreConfirm/13(LM_LR_Line06_fCamValid)
  LM_LR_Line04_dDisStart/1 -> TOS_HWA_CurrentLaneFront_TargPreConfirm/19(LM_LR_Line04_dDisStart)
  LM_LR_Line04_dDisEnd/1 -> TOS_HWA_CurrentLaneFront_TargPreConfirm/20(LM_LR_Line04_dDisEnd)
  LM_LR_Line05_dDisStart/1 -> TOS_HWA_CurrentLaneFront_TargPreConfirm/21(LM_LR_Line05_dDisStart)
  LM_LR_Line05_dDisEnd/1 -> TOS_HWA_CurrentLaneFront_TargPreConfirm/22(LM_LR_Line05_dDisEnd)
  LM_LR_Line06_dDisStart/1 -> TOS_HWA_CurrentLaneFront_TargPreConfirm/23(LM_LR_Line06_dDisStart)
  LM_LR_Line06_dDisEnd/1 -> TOS_HWA_CurrentLaneFront_TargPreConfirm/24(LM_LR_Line06_dDisEnd)
  TOS_HWA_CurrentLaneFront_TargPreConfirm/1(TOS_HWA_TargetPre_Filt_Flag) -> Merge/1
  TOS_HWA_CurrentLaneFront_TargPreConfirm/2(TOS_HWA_TargetPre_1_ConditionFlag_ObserVale) -> Merge1/1
  TOS_HWA_CurrentLaneFront_TargPreConfirm/3(TOS_HWA_TargetPre_FusionTypeFlag_ObserVale) -> Merge2/1
  TOS_HWA_CurrentLaneFront_TargPreConfirm/4(TOS_HWA_TargetPre_PassedbyTarget_Flag_ObserVale) -> Merge3/1
  TOS_HWA_CurrentLaneFront_TargPreConfirm/5(TOS_HWA_TargetPre_FenceFlag_ObserVale) -> Merge4/1
  TOS_HWA_CurrentLaneFront_TargPreConfirm/6(TOS_HWA_TargetPre_ObjType_ObserVale) -> Merge5/1
  TOS_HWA_CurrentLaneFront_TargPreConfirm/7(TOS_HWA_TargetPre_OverlapThre_Val_ObserVale) -> Merge6/1
  TOS_HWA_CurrentLaneFront_TargPreConfirm/8(TOS_HWA_TargetPre_SameLane_Flag) -> Merge9/1
  TOS_HWA_CurrentLaneFront_TargPreConfirm/9(TOS_HWA_TargetPre_2_OverlapThre_ObserVale) -> Merge7/1
  TOS_HWA_CurrentLaneFront_TargPreConfirm/10(TOS_HWA_TargetPre_3_SameLane_Flag_ObserVale) -> Merge8/1
  [Obj_Dx] -> Compare To Constant2/1, Compare To Constant1/1
  Compare To Constant1/1 -> Logical Operator3/2
  Logical Operator3/1 -> If/1
  Compare To Constant2/1 -> Logical Operator1/2
  Logical Operator1/1 -> If/2
  If/2 -> TOS_HWA_CurrentLaneRear_TargPreConfirmDefault/Action
  If/3 -> Default/Action
  Merge3/1 -> TOS_HWA_TargetPre_PassedbyTarget_Flag_ObserVale/1
  Merge8/1 -> TOS_HWA_TargetPre_3_SameLane_Flag_ObserVale/1
  Merge5/1 -> TOS_HWA_TargetPre_ObjType_ObserVale/1
  Merge4/1 -> TOS_HWA_TargetPre_FenceFlag_ObserVale/1
  Merge9/1 -> TOS_HWA_TargetPre_SameLane_Flag/1
  Merge/1 -> TOS_HWA_TargetPre_Filt_Flag/1
  Merge2/1 -> TOS_HWA_TargetPre_FusionTypeFlag_ObserVale/1
  Merge7/1 -> TOS_HWA_TargetPre_2_OverlapThre_ObserVale/1
  Merge1/1 -> TOS_HWA_TargetPre_1_ConditionFlag_ObserVale/1
  Merge6/1 -> TOS_HWA_TargetPre_OverlapThre_Val_ObserVale/1
  TOS_HWA_CurrentLaneRear_TargPreConfirmDefault/10(TOS_HWA_TargetPre_3_SameLane_Flag_ObserVale) -> Merge8/2
  TOS_HWA_CurrentLaneRear_TargPreConfirmDefault/9(TOS_HWA_TargetPre_2_OverlapThre_ObserVale) -> Merge7/2
  TOS_HWA_CurrentLaneRear_TargPreConfirmDefault/8(TOS_HWA_TargetPre_SameLane_Flag) -> Merge9/2
  TOS_HWA_CurrentLaneRear_TargPreConfirmDefault/7(TOS_HWA_TargetPre_OverlapThre_Val_ObserVale) -> Merge6/2
  TOS_HWA_CurrentLaneRear_TargPreConfirmDefault/6(TOS_HWA_TargetPre_ObjType_ObserVale) -> Merge5/2
  TOS_HWA_CurrentLaneRear_TargPreConfirmDefault/5(TOS_HWA_TargetPre_FenceFlag_ObserVale) -> Merge4/2
  TOS_HWA_CurrentLaneRear_TargPreConfirmDefault/4(TOS_HWA_TargetPre_PassedbyTarget_Flag_ObserVale) -> Merge3/2
  TOS_HWA_CurrentLaneRear_TargPreConfirmDefault/3(TOS_HWA_TargetPre_FusionTypeFlag_ObserVale) -> Merge2/2
  TOS_HWA_CurrentLaneRear_TargPreConfirmDefault/2(TOS_HWA_TargetPre_1_ConditionFlag_ObserVale) -> Merge1/2
  TOS_HWA_CurrentLaneRear_TargPreConfirmDefault/1(TOS_HWA_TargetPre_Filt_Flag) -> Merge/2
  Default/10(TOS_HWA_TargetPre_3_SameLane_Flag_ObserVale) -> Merge8/3
  Default/9(TOS_HWA_TargetPre_2_OverlapThre_ObserVale) -> Merge7/3
  Default/8(TOS_HWA_TargetPre_SameLane_Flag) -> Merge9/3
  Default/7(TOS_HWA_TargetPre_OverlapThre_Val_ObserVale) -> Merge6/3
  Default/6(TOS_HWA_TargetPre_ObjType_ObserVale) -> Merge5/3
  Default/5(TOS_HWA_TargetPre_FenceFlag_ObserVale) -> Merge4/3
  Default/4(TOS_HWA_TargetPre_PassedbyTarget_Flag_ObserVale) -> Merge3/3
  Default/3(TOS_HWA_TargetPre_FusionTypeFlag_ObserVale) -> Merge2/3
  Default/2(TOS_HWA_TargetPre_1_ConditionFlag_ObserVale) -> Merge1/3
  Default/1(TOS_HWA_TargetPre_Filt_Flag) -> Merge/3

== system PubIfDecisionTOS_MDL/TOS_20201112/TOS_2012080320/TOS/LC_LCKie_ELK/TOS_HWA/LeftLane/HWA_Object_PreConfirm/HWA_Object_PreConfirm ==
  PP_ObjFusType_FC_FR_Confirm : Inport  Partition=on  PartitionDimension=1  PartitionWidth=1  PartitionOffset=0
  PP_ObjFusType_FR_Confirm : Inport  Port=2  Partition=on  PartitionDimension=1  PartitionWidth=1  PartitionOffset=0
  PP_ObjFusType_FC_Confirm : Inport  Port=3  Partition=on  PartitionDimension=1  PartitionWidth=1  PartitionOffset=0
  Object_ID : Inport  Port=4  OutDataTypeStr=uint8  Partition=on  PartitionDimension=1  PartitionWidth=1  PartitionOffset=0
  Obj_MovingState : Inport  Port=5  Partition=on  PartitionDimension=1  PartitionWidth=1  PartitionOffset=0
  Obj_Dx : Inport  Port=6  Partition=on  PartitionDimension=1  PartitionWidth=1  PartitionOffset=0
  Object_ObstacleProb : Inport  Port=7  Partition=on  PartitionDimension=1  PartitionWidth=1  PartitionOffset=0
  Object_DY : Inport  Port=8  Partition=on  PartitionDimension=1  PartitionWidth=1  PartitionOffset=0
  Object_ObjType : Inport  Port=9  Partition=on  PartitionDimension=1  PartitionWidth=1  PartitionOffset=0
  Compare To Constant : simulink/Logic and Bit Operations/Compare To Constant  relop=~=  const=C_TOS_OFMObjIDInvilad_Val  OutDataTypeStr=boolean
      settings: AttributesFormatString=C_TOS_OFMObjIDInvilad_Val = 0
  Compare To Constant1 : simulink/Logic and Bit Operations/Compare To Constant  relop=>=  const=single(7)  OutDataTypeStr=boolean
      settings: AttributesFormatString=dx >= single(0)
  Compare To Constant2 : simulink/Logic and Bit Operations/Compare To Constant  relop=<  const=single(7)  OutDataTypeStr=boolean
      settings: AttributesFormatString=dx >= single(0)
  Default : Subsystem  TreatAsAtomicUnit=on
  For Each : ForEach  DisableCoverage=on
  HWA_Object_PreConfirm : Subsystem
  HWA_Object_PreConfirmDefault1 : Subsystem  TreatAsAtomicUnit=on
  If1 : If  NumInputs=2  IfExpression=u1 == 1  ElseIfExpressions=u2 == 1
  Logical Operator1 : Logic  AllPortsSameDT=off  OutDataTypeStr=boolean
  Logical Operator3 : Logic  AllPortsSameDT=off  OutDataTypeStr=boolean
  Merge{,1,3..5} (5 alike) : Merge  Inputs=3
  TOS_HWA_TargetPre_Confirm_Filt_Flag : Outport  ConcatenationDimension=1
  TOS_HWA_TargetPre_FusionTypeFlag_ObserVale : Outport  Port=2  ConcatenationDimension=1
  TOS_HWA_TargetPre_PassedbyTarget_ObserVale : Outport  Port=3  ConcatenationDimension=1
  TOS_HWA_TargetPre_ObjType_ObserVale : Outport  Port=4  ConcatenationDimension=1
  TOS_HWA_DyConfirm_ObserVale : Outport  Port=5  ConcatenationDimension=1
  wires:
  PP_ObjFusType_FC_FR_Confirm/1 -> HWA_Object_PreConfirm/2(PP_ObjFusType_FC_FR_Confirm)
  PP_ObjFusType_FR_Confirm/1 -> HWA_Object_PreConfirm/3(PP_ObjFusType_FR_Confirm)
  Compare To Constant/1 -> Logical Operator1/1, Logical Operator3/1
  Object_ID/1 -> [Object_ID], Compare To Constant/1
  If1/3 -> Default/Action
  If1/1 -> HWA_Object_PreConfirm/Action
  PP_ObjFusType_FC_Confirm/1 -> HWA_Object_PreConfirm/4(PP_ObjFusType_FC_Confirm)
  Obj_MovingState/1 -> HWA_Object_PreConfirm/5(Obj_MovingState)
  Obj_Dx/1 -> HWA_Object_PreConfirm/6(Obj_Dx)
  Object_ObstacleProb/1 -> HWA_Object_PreConfirm/7(Object_ObstacleProb)
  Object_DY/1 -> HWA_Object_PreConfirm/8(Object_DY)
  [Object_ID] -> HWA_Object_PreConfirm/1(Object_ID)
  Object_ObjType/1 -> HWA_Object_PreConfirm/9(Object_ObjType)
  HWA_Object_PreConfirm/1(TOS_HWA_TargetPre_Confirm_Filt_Flag) -> Merge/2
  HWA_Object_PreConfirm/2(TOS_HWA_TargetPre_FusionTypeFlag_ObserVale) -> Merge5/2
  HWA_Object_PreConfirm/3(TOS_HWA_TargetPre_PassedbyTarget_Flag_ObserVale) -> Merge1/2
  HWA_Object_PreConfirm/4(TOS_HWA_TargetPre_ObjType_ObserVale) -> Merge3/2
  HWA_Object_PreConfirm/5(TOS_HWA_DyConfirm_ObserVale) -> Merge4/2
  Merge/1 -> TOS_HWA_TargetPre_Confirm_Filt_Flag/1
  Merge5/1 -> TOS_HWA_TargetPre_FusionTypeFlag_ObserVale/1
  Merge1/1 -> TOS_HWA_TargetPre_PassedbyTarget_ObserVale/1
  Merge3/1 -> TOS_HWA_TargetPre_ObjType_ObserVale/1
  Merge4/1 -> TOS_HWA_DyConfirm_ObserVale/1
  [Obj_Dx] -> Compare To Constant1/1, Compare To Constant2/1
  Compare To Constant1/1 -> Logical Operator3/2
  Compare To Constant2/1 -> Logical Operator1/2
  Logical Operator3/1 -> If1/1
  Logical Operator1/1 -> If1/2
  If1/2 -> HWA_Object_PreConfirmDefault1/Action
  HWA_Object_PreConfirmDefault1/1(TOS_HWA_TargetPre_Confirm_Filt_Flag) -> Merge/1
  HWA_Object_PreConfirmDefault1/2(TOS_HWA_TargetPre_FusionTypeFlag_ObserVale) -> Merge5/1
  HWA_Object_PreConfirmDefault1/3(TOS_HWA_TargetPre_PassedbyTarget_Flag_ObserVale) -> Merge1/1
  HWA_Object_PreConfirmDefault1/4(TOS_HWA_TargetPre_ObjType_ObserVale) -> Merge3/1
  HWA_Object_PreConfirmDefault1/5(TOS_HWA_DyConfirm_ObserVale) -> Merge4/1
  Default/5(TOS_HWA_DyConfirm_ObserVale) -> Merge4/3
  Default/4(TOS_HWA_TargetPre_ObjType_ObserVale) -> Merge3/3
  Default/3(TOS_HWA_TargetPre_PassedbyTarget_Flag_ObserVale) -> Merge1/3
  Default/2(TOS_HWA_TargetPre_FusionTypeFlag_ObserVale) -> Merge5/3
  Default/1(TOS_HWA_TargetPre_Confirm_Filt_Flag) -> Merge/3

== system PubIfDecisionTOS_MDL/TOS_20201112/TOS_2012080320/TOS/LC_LCKie_ELK/TOS_HWA/LeftLane/TOS_HWA_LeftLane/TOS_HWA_LeftLane ==
  HLeftLane_ObjIndex : Inport  Partition=on  PartitionDimension=1  PartitionWidth=1  PartitionOffset=0
  PP_ObjMovingDirSignalProcessing : Inport  Port=2
  Object_VX : Inport  Port=3
  Object_VY : Inport  Port=4
  Object_Type : Inport  Port=5
  Object_MovingState : Inport  Port=6
  TOS_TLJ_LeftLaneConfirm_Flag : Inport  Port=7
  Object_DX : Inport  Port=8
  Object_DY : Inport  Port=9
  Object_Fus_Type : Inport  Port=10
  Object_HeadingAngle : Inport  Port=11
  PP_ObjFusType_FC_FR_Confirm : Inport  Port=12
  PP_ObjFusType_FR_Confirm : Inport  Port=13
  PP_ObjFusType_FC_Confirm : Inport  Port=14
  VIE_EgoVelocity : Inport  Port=15
  Compare To Constant : simulink/Logic and Bit Operations/Compare To Constant  relop===  const=C_TOS_OFMObjIDInvilad_Val  OutDataTypeStr=boolean
      settings: AttributesFormatString=C_TOS_OFMObjIDInvilad_Val = 0
  Constant : Constant  Value=0  OutDataTypeStr=uint8
  Constant1 : Constant  Value=0  OutDataTypeStr=uint8
  Constant2 : Constant  Value=0  OutDataTypeStr=uint8
  Constant3 : Constant  Value=C_TOS_ObjInLeftLaneValid  OutDataTypeStr=uint8
      settings: AttributesFormatString=C_TOS_ObjInLeftLaneValid = 2
  For Each : ForEach  DisableCoverage=on
  If : If  IfExpression=u1 ~= 0
  Merge{1..11} (11 alike) : Merge
  Switch : Switch  Criteria=u2 ~= 0
  Switch1 : Switch  Criteria=u2 ~= 0
  Switch2 : Switch  Criteria=u2 ~= 0
  TOS_HWA : Subsystem
  TOS_HWA_Default : Subsystem  TreatAsAtomicUnit=on
  TOS_HWA_TargetInLeftLane_b : Outport  ConcatenationDimension=1
  TOS_HWA_LeftFront_TargConfirm_b : Outport  Port=2  ConcatenationDimension=1
  TOS_HWA_LeftRear_TargConfirm_b : Outport  Port=3  ConcatenationDimension=1
  TOS_HWA_LeftFront_FusType_ObserVale : Outport  Port=4  ConcatenationDimension=1
  TOS_HWA_InLeftLane_Front_Flag_ObserVale : Outport  Port=5  ConcatenationDimension=1
  TOS_HWA_LeftFront_TargMovDir_ObserVale : Outport  Port=6  ConcatenationDimension=1
  TOS_HWA_LeftRear_MovState_ObserVale : Outport  Port=7  ConcatenationDimension=1
  TOS_HWA_LeftRear_FusionType_ObserVale : Outport  Port=8  ConcatenationDimension=1
  TOS_HWA_InLeftLane_Rear_Flag_ObserVale : Outport  Port=9  ConcatenationDimension=1
  TOS_HWA_LeftRear_TargetMovingDir_ObserVale : Outport  Port=10  ConcatenationDimension=1
  TOS_HWA_LeftRear_DyConfirm_ObserVale : Outport  Port=11  ConcatenationDimension=1
  wires:
  Object_DY/1 -> TOS_HWA/9(Object_DY)  "Object_DY"
  TOS_HWA_Default/11(TOS_HWA_LeftRear_DyConfirm_ObserVale) -> Merge11/1
  TOS_HWA_Default/10(TOS_HWA_LeftRear_TargetMovingDir_ObserVale) -> Merge10/1
  TOS_HWA_Default/9(TOS_HWA_InLeftLane_Rear_Flag_ObserVale) -> Merge9/1
  TOS_HWA_Default/8(TOS_HWA_LeftRear_FusionType_ObserVale) -> Merge8/1
  TOS_HWA_Default/7(TOS_HWA_LeftRear_MovState_ObserVale) -> Merge7/1
  TOS_HWA_Default/6(TOS_HWA_LeftFront_TargMovDir_ObserVale) -> Merge6/1
  TOS_HWA_Default/5(TOS_HWA_InLeftLane_Front_Flag_ObserVale) -> Merge2/1
  TOS_HWA_Default/4(TOS_HWA_LeftFront_FusType_ObserVale) -> Merge1/1
  Merge10/1 -> TOS_HWA_LeftRear_TargetMovingDir_ObserVale/1
  Merge9/1 -> TOS_HWA_InLeftLane_Rear_Flag_ObserVale/1
  Merge8/1 -> TOS_HWA_LeftRear_FusionType_ObserVale/1
  Merge7/1 -> TOS_HWA_LeftRear_MovState_ObserVale/1
  Merge6/1 -> TOS_HWA_LeftFront_TargMovDir_ObserVale/1
  Merge2/1 -> TOS_HWA_InLeftLane_Front_Flag_ObserVale/1
  Merge11/1 -> TOS_HWA_LeftRear_DyConfirm_ObserVale/1
  Merge1/1 -> TOS_HWA_LeftFront_FusType_ObserVale/1
  Merge3/1 -> Switch2/2
  TOS_HWA_Default/3(TOS_HWA_LeftRear_TargConfirm_b) -> Merge5/1
  TOS_HWA_Default/2(TOS_HWA_LeftFront_TargConfirm_b) -> Merge4/1
  Merge5/1 -> Switch1/2
  Merge4/1 -> Switch/2
  TOS_HWA_Default/1(TOS_HWA_TargetInLeftLane_b) -> Merge3/1
  TOS_HWA/10(TOS_HWA_LeftRear_TargetMovingDir_ObserVale) -> Merge10/2
  TOS_HWA/9(TOS_HWA_InLeftLane_Rear_Flag_ObserVale) -> Merge9/2
  TOS_HWA/8(TOS_HWA_LeftRear_FusionType_ObserVale) -> Merge8/2
  TOS_HWA/7(TOS_HWA_LeftRear_MovState_ObserVale) -> Merge7/2
  TOS_HWA/6(TOS_HWA_LeftFront_TargMovDir_ObserVale) -> Merge6/2
  TOS_HWA/5(TOS_HWA_InLeftLane_Front_Flag_ObserVale) -> Merge2/2
  TOS_HWA/4(TOS_HWA_LeftFront_FusType_ObserVale) -> Merge1/2
  TOS_HWA/3(TOS_HWA_LeftRear_TargConfirm_b) -> Merge5/2
  TOS_HWA/2(TOS_HWA_LeftFront_TargConfirm_b) -> Merge4/2
  TOS_HWA/1(TOS_HWA_TargetInLeftLane_b) -> Merge3/2
  TOS_HWA/11(TOS_HWA_LeftRear_DyConfirm_ObserVale) -> Merge11/2
  VIE_EgoVelocity/1 -> TOS_HWA/15(VIE_EgoVelocity)
  PP_ObjFusType_FR_Confirm/1 -> TOS_HWA/13(PP_ObjFusType_FR_Confirm)
  PP_ObjFusType_FC_FR_Confirm/1 -> TOS_HWA/12(PP_ObjFusType_FC_FR_Confirm)
  PP_ObjFusType_FC_Confirm/1 -> TOS_HWA/14(PP_ObjFusType_FC_Confirm)
  Switch2/1 -> TOS_HWA_TargetInLeftLane_b/1
  Constant2/1 -> Switch2/3
  Constant3/1 -> Switch2/1
  [HWA_LeftLane_ObjIndex] -> TOS_HWA/1(HWA_LeftLane_ObjIndex)
  [HWA_LeftLane_ObjIndex] -> Switch1/1
  Constant1/1 -> Switch1/3
  Switch1/1 -> TOS_HWA_LeftRear_TargConfirm_b/1
  Switch/1 -> TOS_HWA_LeftFront_TargConfirm_b/1
  Constant/1 -> Switch/3
  [HWA_LeftLane_ObjIndex] -> Switch/1
  HLeftLane_ObjIndex/1 -> Compare To Constant/1, [HWA_LeftLane_ObjIndex]
  Object_HeadingAngle/1 -> TOS_HWA/11(Object_HeadingAngle)  "Object_HeadingAngle"
  Object_Fus_Type/1 -> TOS_HWA/10(Object_Fus_Type)
  Object_DX/1 -> TOS_HWA/8(Object_DX)  "Object_DX"
  TOS_TLJ_LeftLaneConfirm_Flag/1 -> TOS_HWA/7(TOS_TLJ_LeftLaneConfirm_Flag)
  Object_MovingState/1 -> TOS_HWA/6(object_MovingState)
  Object_Type/1 -> TOS_HWA/5(Object_Type)
  Object_VY/1 -> TOS_HWA/4(Object_VY)
  Object_VX/1 -> TOS_HWA/3(Object_VX)
  PP_ObjMovingDirSignalProcessing/1 -> TOS_HWA/2(PP_ObjMovingDirSignalProcessing)
  If/2 -> TOS_HWA/Action
  Compare To Constant/1 -> If/1
  If/1 -> TOS_HWA_Default/Action
